simulink model "swapnil"  (R2018b)
settings: Solver=VariableStepAuto  StartTime=0.0  StopTime=10.0  RelTol=1e-3
settings Model: Creator=student  LastModifiedBy=pal35

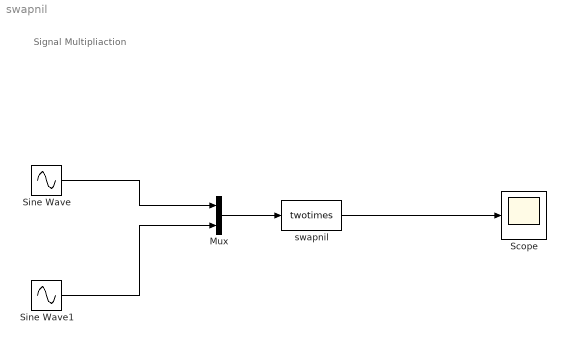
== system swapnil ==
  note: Signal Multipliaction
  Mux : Mux  Inputs=2
  Scope : Scope
  Sine Wave : Sin  SampleTime=0
  Sine Wave1 : Sin  Amplitude=2  SampleTime=0
  swapnil : S-Function  FunctionName=twotimes  Parameters=5  SFunctionDeploymentMode=off  EnableBusSupport=off
  wires:
  Sine Wave/1 -> Mux/1
  Sine Wave1/1 -> Mux/2
  Mux/1 -> swapnil/1
  swapnil/1 -> Scope/1
